simulink model "PID"  (R2020b)
settings: Solver=VariableStepAuto  StartTime=0.0  StopTime=10.0  RelTol=1e-3
model workspace (MAT data in the model file):
  Kd = 0.20397
  Ki = 400
  Kp = 22.586
  N = 79169.4921
settings Model: Creator=user  LastModifiedBy=user

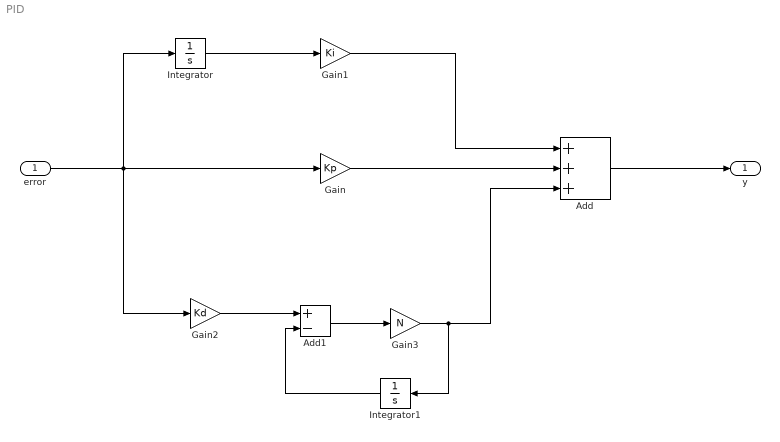
== system PID ==
  error : Inport  OutDataTypeStr=double  PortDimensions=1  SampleTime=0
  Add : Sum  Inputs=+++
  Add1 : Sum  Inputs=+-
  Gain : Gain  Gain=Kp
  Gain1 : Gain  Gain=Ki
  Gain2 : Gain  Gain=Kd
  Gain3 : Gain  Gain=N
  Integrator : Integrator
  Integrator1 : Integrator
  y : Outport  OutDataTypeStr=double  PortDimensions=1  SampleTime=0
  wires:
  Gain/1 -> Add/2
  Add/1 -> y/1
  Integrator/1 -> Gain1/1
  Gain2/1 -> Add1/1
  Integrator1/1 -> Add1/2
  Add1/1 -> Gain3/1
  Gain3/1 -> Integrator1/1, Add/3
  error/1 -> Gain2/1, Gain/1, Integrator/1
  Gain1/1 -> Add/1
